simulink library "HEMERO"  (Simulink 3.00)
values from neighbouring files (symbols this model uses):
  K1 = 0.5    [ejh64.m]    (also in ejh65.m)
  K2 = 0.8    [ejh64.m]    (also in ejh65.m)
  x_camino = 0:0.01:10    [ejh64.m]    (also in ejh65.m)
  y_camino = x_camino.^2    [ejh64.m]    (also in ejh65.m)
undefined symbols (not defined in the file or in its folder): magnitude, nonlinear
libraries: simulink_extras x12, HEMERO x9, simulink3 x6, dspstat x4
(part 5 of 9)

== system HEMERO/Robots móviles/Control de robots móviles/Métodos basados en Teoría de Control/Seguimiento de caminos/Seguimiento de caminos (control lineal)/Convertidor ==
  R_c : Inport  Port=1  PortWidth=-1  SampleTime=-1  DataType=auto
      settings: SignalType=auto
  fi_gorro : Inport  Port=2  PortWidth=-1  SampleTime=-1  DataType=auto
      settings: SignalType=auto
  v : Inport  Port=3  PortWidth=-1  SampleTime=-1  DataType=auto
      settings: SignalType=auto
  u_cont : Inport  Port=4  PortWidth=-1  SampleTime=-1  DataType=auto
      settings: SignalType=auto
  Constant : Constant  Value=1
  Gain : Gain  Gain=-1  SaturateOnIntegerOverflow=on
  Math Function : Math  Operator=reciprocal  OutputSignalType=auto
  Math Function1 : Math  Operator=reciprocal  OutputSignalType=auto
  Product : Product  Inputs=3  SaturateOnIntegerOverflow=on
  Product1 : Product  Inputs=3  SaturateOnIntegerOverflow=on
  Product2 : Product  Inputs=2  SaturateOnIntegerOverflow=on
  Sum : Sum  Inputs=++  SaturateOnIntegerOverflow=on
  Sum1 : Sum  Inputs=++  SaturateOnIntegerOverflow=on
  Trigonometric Function : Trigonometry  Operator=cos  OutputSignalType=auto
  Trigonometric Function1 : Trigonometry  Operator=sin  OutputSignalType=auto
  w : Outport  Port=1  InitialOutput=0
  wires:
  Product2/1 -> Product/3
  Sum/1 -> w/1
  u_cont/1 -> Sum/1
  Product/1 -> Sum/2
  Math Function/1 -> Product2/1
  v/1 -> Product/2, Product1/2
  Trigonometric Function/1 -> Product/1
  Sum1/1 -> Math Function/1
  Constant/1 -> Sum1/2
  Product1/1 -> Sum1/1
  Gain/1 -> Product1/3
  Trigonometric Function1/1 -> Product1/1
  fi_gorro/1 -> Trigonometric Function1/1, Trigonometric Function/1
  R_c/1 -> Math Function1/1
  Math Function1/1 -> Product2/2, Gain/1

== system HEMERO/Robots móviles/Control de robots móviles/Métodos basados en Teoría de Control/Seguimiento de caminos/Seguimiento de caminos (control lineal)/Cálculo de parámetros ==
  x_camino : Inport  Port=1  PortWidth=-1  SampleTime=-1  DataType=auto
      settings: SignalType=auto
  y_camino : Inport  Port=2  PortWidth=-1  SampleTime=-1  DataType=auto
      settings: SignalType=auto
  x_vehiculo : Inport  Port=3  PortWidth=-1  SampleTime=-1  DataType=auto
      settings: SignalType=auto
  y_vehiculo : Inport  Port=4  PortWidth=-1  SampleTime=-1  DataType=auto
      settings: SignalType=auto
  phi_vehiculo : Inport  Port=5  PortWidth=-1  SampleTime=-1  DataType=auto
      settings: SignalType=auto
  Cálculo de phi gorro : Subsystem
  Degrees to Radians : simulink_extras/Transformations/Degrees to Radians
  Subsystem : Subsystem
  epsilon : Outport  Port=1
  fi_gorro : Outport  Port=2
  R_c : Outport  Port=3
  wires:
  Subsystem/2(indice) -> Cálculo de phi gorro/2(indice)
  Subsystem/1(distancia) -> epsilon/1
  Cálculo de phi gorro/1(fi_go_mo) -> Degrees to Radians/1
  Degrees to Radians/1 -> fi_gorro/1
  phi_vehiculo/1 -> Cálculo de phi gorro/1(fi_vehiculo)
  Subsystem/3(R_c) -> R_c/1
  x_vehiculo/1 -> Subsystem/3(x_vehiculo)
  y_vehiculo/1 -> Subsystem/4(y_vehiculo)
  y_camino/1 -> Subsystem/2(y_camino)
  x_camino/1 -> Subsystem/1(x_camino)

== system HEMERO/Robots móviles/Control de robots móviles/Métodos basados en Teoría de Control/Seguimiento de caminos/Seguimiento de caminos (control no lineal)/  ==
  v : Inport  Port=1  PortWidth=-1  SampleTime=-1  DataType=auto
      settings: SignalType=auto
  Abs : Abs
  Gain : Gain  Gain=K2  SaturateOnIntegerOverflow=on
  k (v) : Outport  Port=1
  wires:
  Gain/1 -> k (v)/1
  Abs/1 -> Gain/1
  v/1 -> Abs/1

== system HEMERO/Robots móviles/Control de robots móviles/Métodos basados en Teoría de Control/Seguimiento de caminos/Seguimiento de caminos (control no lineal)/Configuracion síncrona ==
  v : Inport  Port=1  PortWidth=-1  SampleTime=-1  DataType=auto
      settings: SignalType=auto
  w : Inport  Port=2  PortWidth=-1  SampleTime=-1  DataType=auto
      settings: SignalType=auto
  Fcn : Fcn  Expr=-sin(u)
  Fcn1 : Fcn  Expr=cos(u)
  Integrator : Integrator  ExternalReset=none  InitialConditionSource=internal  InitialCondition=phi_inicial  LimitOutput=off  UpperSaturationLimit=inf  LowerSaturationLimit=-inf  ShowSaturationPort=off  ShowStatePort=off  AbsoluteTolerance=auto
  Integrator1 : Integrator  ExternalReset=none  InitialConditionSource=internal  InitialCondition=x_inicial  LimitOutput=off  UpperSaturationLimit=inf  LowerSaturationLimit=-inf  ShowSaturationPort=off  ShowStatePort=off  AbsoluteTolerance=auto
  Integrator2 : Integrator  ExternalReset=none  InitialConditionSource=internal  InitialCondition=y_inicial  LimitOutput=off  UpperSaturationLimit=inf  LowerSaturationLimit=-inf  ShowSaturationPort=off  ShowStatePort=off  AbsoluteTolerance=auto
  Product : Product  Inputs=2  SaturateOnIntegerOverflow=on
  Product1 : Product  Inputs=2  SaturateOnIntegerOverflow=on
  x_vehículo : Outport  Port=1
  y_vehículo : Outport  Port=2
  phi_vehículo : Outport  Port=3
  wires:
  Fcn1/1 -> Product1/2
  w/1 -> Integrator/1
  v/1 -> Product1/1, Product/1
  Integrator2/1 -> y_vehículo/1
  Integrator1/1 -> x_vehículo/1
  Integrator/1 -> phi_vehículo/1, Fcn1/1, Fcn/1
  Fcn/1 -> Product/2
  Product/1 -> Integrator1/1
  Product1/1 -> Integrator2/1

== system HEMERO/Robots móviles/Control de robots móviles/Métodos basados en Teoría de Control/Seguimiento de caminos/Seguimiento de caminos (control no lineal)/Controlador no lineal ==
  phi_gorro : Inport  Port=1  PortWidth=-1  SampleTime=-1  DataType=auto
      settings: SignalType=auto
  v : Inport  Port=2  PortWidth=-1  SampleTime=-1  DataType=auto
      settings: SignalType=auto
  epsilon : Inport  Port=3  PortWidth=-1  SampleTime=-1  DataType=auto
      settings: SignalType=auto
  k (v) : Inport  Port=4  PortWidth=-1  SampleTime=-1  DataType=auto
      settings: SignalType=auto
  Gain : Gain  Gain=K1  SaturateOnIntegerOverflow=on
  MATLAB Fcn : MATLABFcn  MATLABFcn=nonlinear(u)  OutputWidth=-1  OutputSignalType=auto
  Product : Product  Inputs=3  SaturateOnIntegerOverflow=on
  Product1 : Product  Inputs=2  SaturateOnIntegerOverflow=on
  Sum : Sum  Inputs=--  SaturateOnIntegerOverflow=on
  u_cont : Outport  Port=1  InitialOutput=0
  wires:
  k (v)/1 -> Product1/2
  v/1 -> Product/2
  phi_gorro/1 -> Product1/1, MATLAB Fcn/1
  Gain/1 -> Product/1
  Product/1 -> Sum/1
  Product1/1 -> Sum/2
  epsilon/1 -> Gain/1
  Sum/1 -> u_cont/1
  MATLAB Fcn/1 -> Product/3

== system HEMERO/Robots móviles/Control de robots móviles/Métodos basados en Teoría de Control/Seguimiento de caminos/Seguimiento de caminos (control no lineal)/Convertidor ==
  R_c : Inport  Port=1  PortWidth=-1  SampleTime=-1  DataType=auto
      settings: SignalType=auto
  fi_gorro : Inport  Port=2  PortWidth=-1  SampleTime=-1  DataType=auto
      settings: SignalType=auto
  v : Inport  Port=3  PortWidth=-1  SampleTime=-1  DataType=auto
      settings: SignalType=auto
  u_cont : Inport  Port=4  PortWidth=-1  SampleTime=-1  DataType=auto
      settings: SignalType=auto
  Constant : Constant  Value=1
  Gain : Gain  Gain=-1  SaturateOnIntegerOverflow=on
  Math Function : Math  Operator=reciprocal  OutputSignalType=auto
  Math Function1 : Math  Operator=reciprocal  OutputSignalType=auto
  Product : Product  Inputs=3  SaturateOnIntegerOverflow=on
  Product1 : Product  Inputs=3  SaturateOnIntegerOverflow=on
  Product2 : Product  Inputs=2  SaturateOnIntegerOverflow=on
  Sum : Sum  Inputs=++  SaturateOnIntegerOverflow=on
  Sum1 : Sum  Inputs=++  SaturateOnIntegerOverflow=on
  Trigonometric Function : Trigonometry  Operator=cos  OutputSignalType=auto
  Trigonometric Function1 : Trigonometry  Operator=sin  OutputSignalType=auto
  w : Outport  Port=1  InitialOutput=0
  wires:
  Math Function1/1 -> Gain/1, Product2/2
  R_c/1 -> Math Function1/1
  fi_gorro/1 -> Trigonometric Function/1, Trigonometric Function1/1
  Trigonometric Function1/1 -> Product1/1
  Gain/1 -> Product1/3
  Product1/1 -> Sum1/1
  Constant/1 -> Sum1/2
  Sum1/1 -> Math Function/1
  Trigonometric Function/1 -> Product/1
  v/1 -> Product1/2, Product/2
  Math Function/1 -> Product2/1
  Product/1 -> Sum/2
  u_cont/1 -> Sum/1
  Sum/1 -> w/1
  Product2/1 -> Product/3

== system HEMERO/Robots móviles/Control de robots móviles/Métodos basados en Teoría de Control/Seguimiento de caminos/Seguimiento de caminos (control no lineal)/Cálculo de parámetros ==
  x_camino : Inport  Port=1  PortWidth=-1  SampleTime=-1  DataType=auto
      settings: SignalType=auto
  y_camino : Inport  Port=2  PortWidth=-1  SampleTime=-1  DataType=auto
      settings: SignalType=auto
  x_vehiculo : Inport  Port=3  PortWidth=-1  SampleTime=-1  DataType=auto
      settings: SignalType=auto
  y_vehiculo : Inport  Port=4  PortWidth=-1  SampleTime=-1  DataType=auto
      settings: SignalType=auto
  phi_vehiculo : Inport  Port=5  PortWidth=-1  SampleTime=-1  DataType=auto
      settings: SignalType=auto
  Cálculo de phi gorro : Subsystem
  Degrees to Radians : simulink_extras/Transformations/Degrees to Radians
  Subsystem : Subsystem
  epsilon : Outport  Port=1
  fi_gorro : Outport  Port=2
  R_c : Outport  Port=3
  wires:
  x_camino/1 -> Subsystem/1(x_camino)
  y_camino/1 -> Subsystem/2(y_camino)
  y_vehiculo/1 -> Subsystem/4(y_vehiculo)
  x_vehiculo/1 -> Subsystem/3(x_vehiculo)
  Subsystem/3(R_c) -> R_c/1
  phi_vehiculo/1 -> Cálculo de phi gorro/1(fi_vehiculo)
  Degrees to Radians/1 -> fi_gorro/1
  Cálculo de phi gorro/1(fi_go_mo) -> Degrees to Radians/1
  Subsystem/1(distancia) -> epsilon/1
  Subsystem/2(indice) -> Cálculo de phi gorro/2(indice)

== system HEMERO/Robots móviles/Control de robots móviles/Métodos basados en Teoría de Control/Seguimiento de trayectorias/Ejemplos/Ejemplo H.6.6 ==
  Seguimiento de trayectorias (Control lineal) : Subsystem  mask(Seguimiento de trayectorias empleando una ley de control lineal){K1=1, K2=2, K3=4, x_inicial=1, y_inicial=0.5, phi_inicial=pi/6, x_r_inicial=0, y_r_inicial=0, phi_r_inicial=0}
      mask prompts: K1 "Parámetro K1:"; K2 "Parámetro K2:"; K3 "Parámetro K3:"; x_inicial "Coordenada x inicial del robot:"; y_inicial "Coordenada y inicial del robot:"; phi_inicial "Valor inicial de la orientación del robot (rad):"; x_r_inicial "Coordenada x inicial de la referencia:"; y_r_inicial "Coordenada y inicial de la referencia:"; phi_r_inicial "Orientación inicial de la referencia (rad):"
      mask help:
      | Este bloque permite simular una estrategia de control lineal para el seguimiento de trayectorias. A la entrada se dispone de las velocidades lineal y angular de referencia. Se supone un cierto modelo para el vehículo.
      | El usuario puede modificar fácilmente este bloque para introducir como referencia las coordenadas (x,y) y la orientación deseadas.
  Step : Step  Time=0  Before=0  After=0.2  SampleTime=0
  Step1 : Step  Time=0  Before=0  After=0.3  SampleTime=0
  Step2 : Step  Time=20  Before=0  After=-0.1  SampleTime=0
  Step3 : Step  Time=10  Before=0  After=-0.1  SampleTime=0
  Sum : Sum  Inputs=++  SaturateOnIntegerOverflow=on
  Sum1 : Sum  Inputs=++  SaturateOnIntegerOverflow=on
  To Workspace : ToWorkspace  VariableName=v  SampleTime=-1  SaveFormat=Matrix
  To Workspace1 : ToWorkspace  VariableName=w  SampleTime=-1  SaveFormat=Matrix
  To Workspace2 : ToWorkspace  VariableName=v_r  SampleTime=-1  SaveFormat=Matrix
  To Workspace3 : ToWorkspace  VariableName=w_r  SampleTime=-1  SaveFormat=Matrix
  To Workspace4 : ToWorkspace  VariableName=x_r  SampleTime=-1  SaveFormat=Matrix
  To Workspace5 : ToWorkspace  VariableName=x  SampleTime=-1  SaveFormat=Matrix
  To Workspace6 : ToWorkspace  VariableName=y_r  SampleTime=-1  SaveFormat=Matrix
  To Workspace7 : ToWorkspace  VariableName=y  SampleTime=-1  SaveFormat=Matrix
  To Workspace8 : ToWorkspace  VariableName=phi_r  SampleTime=-1  SaveFormat=Matrix
  To Workspace9 : ToWorkspace  VariableName=phi  SampleTime=-1  SaveFormat=Matrix
  wires:
  Step2/1 -> Sum/1
  Step/1 -> Sum/2
  Step1/1 -> Sum1/1
  Step3/1 -> Sum1/2
  Sum1/1 -> To Workspace3/1, Seguimiento de trayectorias (Control lineal)/2(w_r)
  Sum/1 -> To Workspace2/1, Seguimiento de trayectorias (Control lineal)/1(v_r)
  Seguimiento de trayectorias (Control lineal)/1(v) -> To Workspace/1
  Seguimiento de trayectorias (Control lineal)/2(w) -> To Workspace1/1
  Seguimiento de trayectorias (Control lineal)/3(x_ref) -> To Workspace4/1
  Seguimiento de trayectorias (Control lineal)/5(y_ref) -> To Workspace6/1
  Seguimiento de trayectorias (Control lineal)/6(y) -> To Workspace7/1
  Seguimiento de trayectorias (Control lineal)/7(phi_ref) -> To Workspace8/1
  Seguimiento de trayectorias (Control lineal)/4(x) -> To Workspace5/1
  Seguimiento de trayectorias (Control lineal)/8(phi) -> To Workspace9/1

== system HEMERO/Robots móviles/Control de robots móviles/Métodos basados en Teoría de Control/Seguimiento de trayectorias/Ejemplos/Ejemplo H.6.7 ==
  Seguimiento de trayectorias (Control lineal con escalado de velocidad) : Subsystem  mask(Seguimiento de trayectorias (control lineal y escalado en velocidad)){b=13.75, d=0.9, x_inicial=1, y_inicial=0.5, phi_inicial=pi/6, x_r_inicial=0, y_r_inicial=0, phi_r_inicial=0}
      mask prompts: b "Parámetro beta:"; d "Parámetro delta:"; x_inicial "Coordenada x inicial del robot:"; y_inicial "Coordenada y inicial del robot:"; phi_inicial "Valor inicial de la orientación del robot (rad):"; x_r_inicial "Coordenada x inicial de la referencia:"; y_r_inicial "Coordenada y inicial de la referencia:"; phi_r_inicial "Orientación inicial de la referencia (rad):"
      mask help:
      | Este bloque permite simular una estrategia de control lineal con "escalado en velocidad" para el seguimiento de trayectorias. A la entrada se dispone de las velocidades lineal y angular de referencia. Se supone un cierto modelo para el vehículo.
      | El usuario puede modificar fácilmente este bloque para introducir como referencia las coordenadas (x,y) y la orientación deseadas.
  Step : Step  Time=0  Before=0  After=0.2  SampleTime=0
  Step1 : Step  Time=0  Before=0  After=0.3  SampleTime=0
  Step2 : Step  Time=20  Before=0  After=-0.1  SampleTime=0
  Step3 : Step  Time=10  Before=0  After=-0.1  SampleTime=0
  Sum : Sum  Inputs=++  SaturateOnIntegerOverflow=on
  Sum1 : Sum  Inputs=++  SaturateOnIntegerOverflow=on
  To Workspace : ToWorkspace  VariableName=v  SampleTime=-1  SaveFormat=Matrix
  To Workspace1 : ToWorkspace  VariableName=w  SampleTime=-1  SaveFormat=Matrix
  To Workspace2 : ToWorkspace  VariableName=v_r  SampleTime=-1  SaveFormat=Matrix
  To Workspace3 : ToWorkspace  VariableName=w_r  SampleTime=-1  SaveFormat=Matrix
  To Workspace4 : ToWorkspace  VariableName=x_r  SampleTime=-1  SaveFormat=Matrix
  To Workspace5 : ToWorkspace  VariableName=x  SampleTime=-1  SaveFormat=Matrix
  To Workspace6 : ToWorkspace  VariableName=y_r  SampleTime=-1  SaveFormat=Matrix
  To Workspace7 : ToWorkspace  VariableName=y  SampleTime=-1  SaveFormat=Matrix
  To Workspace8 : ToWorkspace  VariableName=phi_r  SampleTime=-1  SaveFormat=Matrix
  To Workspace9 : ToWorkspace  VariableName=phi  SampleTime=-1  SaveFormat=Matrix
  wires:
  Step2/1 -> Sum/1
  Step/1 -> Sum/2
  Step1/1 -> Sum1/1
  Step3/1 -> Sum1/2
  Sum1/1 -> To Workspace3/1, Seguimiento de trayectorias (Control lineal con escalado de velocidad)/2(w_r)
  Sum/1 -> To Workspace2/1, Seguimiento de trayectorias (Control lineal con escalado de velocidad)/1(v_r)
  Seguimiento de trayectorias (Control lineal con escalado de velocidad)/1(v) -> To Workspace/1
  Seguimiento de trayectorias (Control lineal con escalado de velocidad)/2(w) -> To Workspace1/1
  Seguimiento de trayectorias (Control lineal con escalado de velocidad)/3(x_ref) -> To Workspace4/1
  Seguimiento de trayectorias (Control lineal con escalado de velocidad)/5(y_ref) -> To Workspace6/1
  Seguimiento de trayectorias (Control lineal con escalado de velocidad)/6(y) -> To Workspace7/1
  Seguimiento de trayectorias (Control lineal con escalado de velocidad)/7(phi_ref) -> To Workspace8/1
  Seguimiento de trayectorias (Control lineal con escalado de velocidad)/4(x) -> To Workspace5/1
  Seguimiento de trayectorias (Control lineal con escalado de velocidad)/8(phi) -> To Workspace9/1

== system HEMERO/Robots móviles/Control de robots móviles/Métodos basados en Teoría de Control/Seguimiento de trayectorias/Ejemplos/Ejemplo H.6.8 ==
  Seguimiento de trayectorias (Control no lineal) : Subsystem  mask(Seguimiento de trayectorias empleando una ley de control no lineal){b=13.75, d=0.9, K2=19, x_inicial=1, y_inicial=0.5, phi_inicial=pi/6, x_r_inicial=0, y_r_inicial=0, phi_r_inicial=0}
      mask prompts: b "Parámetro beta:"; d "Parámetro delta:"; K2 "Parámetro K2:"; x_inicial "Coordenada x inicial del robot:"; y_inicial "Coordenada y inicial del robot:"; phi_inicial "Valor inicial de la orientación del robot (rad):"; x_r_inicial "Coordenada x inicial de la referencia:"; y_r_inicial "Coordenada y inicial de la referencia:"; phi_r_inicial "Orientación inicial de la referencia (rad):"
      mask help:
      | Este bloque permite simular una estrategia de control no lineal para el seguimiento de trayectorias. A la entrada se dispone de las velocidades lineal y angular de referencia. Se supone un cierto modelo para el vehículo.
      | El usuario puede modificar este bloque para introducir como referencia las coordenadas (x,y) y la orientación deseadas.
  Step : Step  Time=0  Before=0  After=0.2  SampleTime=0
  Step1 : Step  Time=0  Before=0  After=0.3  SampleTime=0
  Step2 : Step  Time=20  Before=0  After=-0.1  SampleTime=0
  Step3 : Step  Time=10  Before=0  After=-0.1  SampleTime=0
  Sum : Sum  Inputs=++  SaturateOnIntegerOverflow=on
  Sum1 : Sum  Inputs=++  SaturateOnIntegerOverflow=on
  To Workspace : ToWorkspace  VariableName=v  SampleTime=-1  SaveFormat=Matrix
  To Workspace1 : ToWorkspace  VariableName=w  SampleTime=-1  SaveFormat=Matrix
  To Workspace2 : ToWorkspace  VariableName=v_r  SampleTime=-1  SaveFormat=Matrix
  To Workspace3 : ToWorkspace  VariableName=w_r  SampleTime=-1  SaveFormat=Matrix
  To Workspace4 : ToWorkspace  VariableName=x_r  SampleTime=-1  SaveFormat=Matrix
  To Workspace5 : ToWorkspace  VariableName=x  SampleTime=-1  SaveFormat=Matrix
  To Workspace6 : ToWorkspace  VariableName=y_r  SampleTime=-1  SaveFormat=Matrix
  To Workspace7 : ToWorkspace  VariableName=y  SampleTime=-1  SaveFormat=Matrix
  To Workspace8 : ToWorkspace  VariableName=phi_r  SampleTime=-1  SaveFormat=Matrix
  To Workspace9 : ToWorkspace  VariableName=phi  SampleTime=-1  SaveFormat=Matrix
  wires:
  Step2/1 -> Sum/1
  Step/1 -> Sum/2
  Step1/1 -> Sum1/1
  Step3/1 -> Sum1/2
  Sum1/1 -> To Workspace3/1, Seguimiento de trayectorias (Control no lineal)/2(w_r)
  Sum/1 -> To Workspace2/1, Seguimiento de trayectorias (Control no lineal)/1(v_r)
  Seguimiento de trayectorias (Control no lineal)/1(v) -> To Workspace/1
  Seguimiento de trayectorias (Control no lineal)/2(w) -> To Workspace1/1
  Seguimiento de trayectorias (Control no lineal)/3(x_ref) -> To Workspace4/1
  Seguimiento de trayectorias (Control no lineal)/5(y_ref) -> To Workspace6/1
  Seguimiento de trayectorias (Control no lineal)/6(y) -> To Workspace7/1
  Seguimiento de trayectorias (Control no lineal)/7(phi_ref) -> To Workspace8/1
  Seguimiento de trayectorias (Control no lineal)/4(x) -> To Workspace5/1
  Seguimiento de trayectorias (Control no lineal)/8(phi) -> To Workspace9/1

== system HEMERO/Robots móviles/Control de robots móviles/Métodos basados en Teoría de Control/Seguimiento de trayectorias/Seguimiento de trayectorias (Control lineal con escalado de velocidad)/Cambio de variable ==
  x_r : Inport  Port=1  PortWidth=-1  SampleTime=-1  DataType=auto
      settings: SignalType=auto
  x : Inport  Port=2  PortWidth=-1  SampleTime=-1  DataType=auto
      settings: SignalType=auto
  y_r : Inport  Port=3  PortWidth=-1  SampleTime=-1  DataType=auto
      settings: SignalType=auto
  y : Inport  Port=4  PortWidth=-1  SampleTime=-1  DataType=auto
      settings: SignalType=auto
  phi_r : Inport  Port=5  PortWidth=-1  SampleTime=-1  DataType=auto
      settings: SignalType=auto
  phi : Inport  Port=6  PortWidth=-1  SampleTime=-1  DataType=auto
      settings: SignalType=auto
  Cálculo de e1 : Subsystem
  Cálculo de e2 : Subsystem
  Cálculo de e3 : Subsystem
  e1 : Outport  Port=1
  e2 : Outport  Port=2
  e3 : Outport  Port=3
  wires:
  Cálculo de e3/1(e3) -> e3/1
  Cálculo de e2/1(e2) -> e2/1
  Cálculo de e1/1(e1) -> e1/1
  phi/1 -> Cálculo de e1/5(phi), Cálculo de e3/2(phi), Cálculo de e2/5(phi)
  phi_r/1 -> Cálculo de e3/1(phi_r)
  y/1 -> Cálculo de e2/4(y), Cálculo de e1/4(y)
  y_r/1 -> Cálculo de e2/3(y_r), Cálculo de e1/3(y_r)
  x/1 -> Cálculo de e2/2(x), Cálculo de e1/2(x)
  x_r/1 -> Cálculo de e2/1(x_r), Cálculo de e1/1(x_r)

== system HEMERO/Robots móviles/Control de robots móviles/Métodos basados en Teoría de Control/Seguimiento de trayectorias/Seguimiento de trayectorias (Control lineal con escalado de velocidad)/Configuración síncrona referencia ==
  v_r : Inport  Port=1  PortWidth=-1  SampleTime=-1  DataType=auto
      settings: SignalType=auto
  w_r : Inport  Port=2  PortWidth=-1  SampleTime=-1  DataType=auto
      settings: SignalType=auto
  Gain : Gain  Gain=-1  SaturateOnIntegerOverflow=on
  Integrator : Integrator  ExternalReset=none  InitialConditionSource=internal  InitialCondition=phi_r_inicial  LimitOutput=off  UpperSaturationLimit=inf  LowerSaturationLimit=-inf  ShowSaturationPort=off  ShowStatePort=off  AbsoluteTolerance=auto
  Integrator1 : Integrator  ExternalReset=none  InitialConditionSource=internal  InitialCondition=x_r_inicial  LimitOutput=off  UpperSaturationLimit=inf  LowerSaturationLimit=-inf  ShowSaturationPort=off  ShowStatePort=off  AbsoluteTolerance=auto
  Integrator2 : Integrator  ExternalReset=none  InitialConditionSource=internal  InitialCondition=y_r_inicial  LimitOutput=off  UpperSaturationLimit=inf  LowerSaturationLimit=-inf  ShowSaturationPort=off  ShowStatePort=off  AbsoluteTolerance=auto
  Product : Product  Inputs=2  SaturateOnIntegerOverflow=on
  Product1 : Product  Inputs=2  SaturateOnIntegerOverflow=on
  Trigonometric Function : Trigonometry  Operator=sin  OutputSignalType=auto
  Trigonometric Function1 : Trigonometry  Operator=cos  OutputSignalType=auto
  x_r : Outport  Port=1
  y_r : Outport  Port=2
  phi_r : Outport  Port=3
  wires:
  Trigonometric Function1/1 -> Product1/2
  Trigonometric Function/1 -> Gain/1
  w_r/1 -> Integrator/1
  v_r/1 -> Product1/1, Product/1
  Integrator2/1 -> y_r/1
  Integrator1/1 -> x_r/1
  Integrator/1 -> phi_r/1, Trigonometric Function1/1, Trigonometric Function/1
  Gain/1 -> Product/2
  Product/1 -> Integrator1/1
  Product1/1 -> Integrator2/1

== system HEMERO/Robots móviles/Control de robots móviles/Métodos basados en Teoría de Control/Seguimiento de trayectorias/Seguimiento de trayectorias (Control lineal con escalado de velocidad)/Configuración síncrona robot real ==
  v : Inport  Port=1  PortWidth=-1  SampleTime=-1  DataType=auto
      settings: SignalType=auto
  w : Inport  Port=2  PortWidth=-1  SampleTime=-1  DataType=auto
      settings: SignalType=auto
  Gain : Gain  Gain=-1  SaturateOnIntegerOverflow=on
  Integrator : Integrator  ExternalReset=none  InitialConditionSource=internal  InitialCondition=phi_inicial  LimitOutput=off  UpperSaturationLimit=inf  LowerSaturationLimit=-inf  ShowSaturationPort=off  ShowStatePort=off  AbsoluteTolerance=auto
  Integrator1 : Integrator  ExternalReset=none  InitialConditionSource=internal  InitialCondition=x_inicial  LimitOutput=off  UpperSaturationLimit=inf  LowerSaturationLimit=-inf  ShowSaturationPort=off  ShowStatePort=off  AbsoluteTolerance=auto
  Integrator2 : Integrator  ExternalReset=none  InitialConditionSource=internal  InitialCondition=y_inicial  LimitOutput=off  UpperSaturationLimit=inf  LowerSaturationLimit=-inf  ShowSaturationPort=off  ShowStatePort=off  AbsoluteTolerance=auto
  Product : Product  Inputs=2  SaturateOnIntegerOverflow=on
  Product1 : Product  Inputs=2  SaturateOnIntegerOverflow=on
  Trigonometric Function : Trigonometry  Operator=sin  OutputSignalType=auto
  Trigonometric Function1 : Trigonometry  Operator=cos  OutputSignalType=auto
  x : Outport  Port=1
  y : Outport  Port=2
  phi : Outport  Port=3
  wires:
  Trigonometric Function1/1 -> Product1/2
  Trigonometric Function/1 -> Gain/1
  w/1 -> Integrator/1
  v/1 -> Product1/1, Product/1
  Integrator2/1 -> y/1
  Integrator1/1 -> x/1
  Integrator/1 -> phi/1, Trigonometric Function1/1, Trigonometric Function/1
  Gain/1 -> Product/2
  Product/1 -> Integrator1/1
  Product1/1 -> Integrator2/1

== system HEMERO/Robots móviles/Control de robots móviles/Métodos basados en Teoría de Control/Seguimiento de trayectorias/Seguimiento de trayectorias (Control lineal con escalado de velocidad)/Control lineal con escalado de velocidad ==
  e1 : Inport  Port=1  PortWidth=-1  SampleTime=-1  DataType=auto
      settings: SignalType=auto
  e2 : Inport  Port=2  PortWidth=-1  SampleTime=-1  DataType=auto
      settings: SignalType=auto
  e3 : Inport  Port=3  PortWidth=-1  SampleTime=-1  DataType=auto
      settings: SignalType=auto
  v_r : Inport  Port=4  PortWidth=-1  SampleTime=-1  DataType=auto
      settings: SignalType=auto
  w_r : Inport  Port=5  PortWidth=-1  SampleTime=-1  DataType=auto
      settings: SignalType=auto
  Cálculo de u1 : Subsystem
  "Cálculo de u2 " : Subsystem
  u1 : Outport  Port=1
  u2 : Outport  Port=2
  wires:
  Cálculo de u1/2(K1) -> "Cálculo de u2 "/4(K3)
  w_r/1 -> Cálculo de u1/3(w_r)
  "Cálculo de u2 "/1(u2) -> u2/1
  Cálculo de u1/1(u1) -> u1/1
  e3/1 -> "Cálculo de u2 "/2(e3)
  e2/1 -> "Cálculo de u2 "/1(e2)
  v_r/1 -> "Cálculo de u2 "/3(v_r), Cálculo de u1/2(v_r)
  e1/1 -> Cálculo de u1/1(e1)

== system HEMERO/Robots móviles/Control de robots móviles/Métodos basados en Teoría de Control/Seguimiento de trayectorias/Seguimiento de trayectorias (Control lineal)/Cambio de variable ==
  x_r : Inport  Port=1  PortWidth=-1  SampleTime=-1  DataType=auto
      settings: SignalType=auto
  x : Inport  Port=2  PortWidth=-1  SampleTime=-1  DataType=auto
      settings: SignalType=auto
  y_r : Inport  Port=3  PortWidth=-1  SampleTime=-1  DataType=auto
      settings: SignalType=auto
  y : Inport  Port=4  PortWidth=-1  SampleTime=-1  DataType=auto
      settings: SignalType=auto
  phi_r : Inport  Port=5  PortWidth=-1  SampleTime=-1  DataType=auto
      settings: SignalType=auto
  phi : Inport  Port=6  PortWidth=-1  SampleTime=-1  DataType=auto
      settings: SignalType=auto
  Cálculo de e1 : Subsystem
  Cálculo de e2 : Subsystem
  Cálculo de e3 : Subsystem
  e1 : Outport  Port=1
  e2 : Outport  Port=2
  e3 : Outport  Port=3
  wires:
  Cálculo de e3/1(e3) -> e3/1
  Cálculo de e2/1(e2) -> e2/1
  Cálculo de e1/1(e1) -> e1/1
  phi/1 -> Cálculo de e1/5(phi), Cálculo de e3/2(phi), Cálculo de e2/5(phi)
  phi_r/1 -> Cálculo de e3/1(phi_r)
  y/1 -> Cálculo de e2/4(y), Cálculo de e1/4(y)
  y_r/1 -> Cálculo de e2/3(y_r), Cálculo de e1/3(y_r)
  x/1 -> Cálculo de e2/2(x), Cálculo de e1/2(x)
  x_r/1 -> Cálculo de e2/1(x_r), Cálculo de e1/1(x_r)

== system HEMERO/Robots móviles/Control de robots móviles/Métodos basados en Teoría de Control/Seguimiento de trayectorias/Seguimiento de trayectorias (Control lineal)/Configuración síncrona referencia ==
  v_r : Inport  Port=1  PortWidth=-1  SampleTime=-1  DataType=auto
      settings: SignalType=auto
  w_r : Inport  Port=2  PortWidth=-1  SampleTime=-1  DataType=auto
      settings: SignalType=auto
  Gain : Gain  Gain=-1  SaturateOnIntegerOverflow=on
  Integrator : Integrator  ExternalReset=none  InitialConditionSource=internal  InitialCondition=phi_r_inicial  LimitOutput=off  UpperSaturationLimit=inf  LowerSaturationLimit=-inf  ShowSaturationPort=off  ShowStatePort=off  AbsoluteTolerance=auto
  Integrator1 : Integrator  ExternalReset=none  InitialConditionSource=internal  InitialCondition=x_r_inicial  LimitOutput=off  UpperSaturationLimit=inf  LowerSaturationLimit=-inf  ShowSaturationPort=off  ShowStatePort=off  AbsoluteTolerance=auto
  Integrator2 : Integrator  ExternalReset=none  InitialConditionSource=internal  InitialCondition=y_r_inicial  LimitOutput=off  UpperSaturationLimit=inf  LowerSaturationLimit=-inf  ShowSaturationPort=off  ShowStatePort=off  AbsoluteTolerance=auto
  Product : Product  Inputs=2  SaturateOnIntegerOverflow=on
  Product1 : Product  Inputs=2  SaturateOnIntegerOverflow=on
  Trigonometric Function : Trigonometry  Operator=sin  OutputSignalType=auto
  Trigonometric Function1 : Trigonometry  Operator=cos  OutputSignalType=auto
  x_r : Outport  Port=1
  y_r : Outport  Port=2
  phi_r : Outport  Port=3
  wires:
  Gain/1 -> Product/2
  Trigonometric Function/1 -> Gain/1
  w_r/1 -> Integrator/1
  v_r/1 -> Product1/1, Product/1
  Integrator2/1 -> y_r/1
  Integrator1/1 -> x_r/1
  Integrator/1 -> phi_r/1, Trigonometric Function/1, Trigonometric Function1/1
  Trigonometric Function1/1 -> Product1/2
  Product/1 -> Integrator1/1
  Product1/1 -> Integrator2/1

== system HEMERO/Robots móviles/Control de robots móviles/Métodos basados en Teoría de Control/Seguimiento de trayectorias/Seguimiento de trayectorias (Control lineal)/Configuración síncrona robot real ==
  v : Inport  Port=1  PortWidth=-1  SampleTime=-1  DataType=auto
      settings: SignalType=auto
  w : Inport  Port=2  PortWidth=-1  SampleTime=-1  DataType=auto
      settings: SignalType=auto
  Gain : Gain  Gain=-1  SaturateOnIntegerOverflow=on
  Integrator : Integrator  ExternalReset=none  InitialConditionSource=internal  InitialCondition=phi_inicial  LimitOutput=off  UpperSaturationLimit=inf  LowerSaturationLimit=-inf  ShowSaturationPort=off  ShowStatePort=off  AbsoluteTolerance=auto
  Integrator1 : Integrator  ExternalReset=none  InitialConditionSource=internal  InitialCondition=x_inicial  LimitOutput=off  UpperSaturationLimit=inf  LowerSaturationLimit=-inf  ShowSaturationPort=off  ShowStatePort=off  AbsoluteTolerance=auto
  Integrator2 : Integrator  ExternalReset=none  InitialConditionSource=internal  InitialCondition=y_inicial  LimitOutput=off  UpperSaturationLimit=inf  LowerSaturationLimit=-inf  ShowSaturationPort=off  ShowStatePort=off  AbsoluteTolerance=auto
  Product : Product  Inputs=2  SaturateOnIntegerOverflow=on
  Product1 : Product  Inputs=2  SaturateOnIntegerOverflow=on
  Trigonometric Function : Trigonometry  Operator=sin  OutputSignalType=auto
  Trigonometric Function1 : Trigonometry  Operator=cos  OutputSignalType=auto
  x : Outport  Port=1
  y : Outport  Port=2
  phi : Outport  Port=3
  wires:
  Trigonometric Function1/1 -> Product1/2
  Trigonometric Function/1 -> Gain/1
  w/1 -> Integrator/1
  v/1 -> Product1/1, Product/1
  Integrator2/1 -> y/1
  Integrator1/1 -> x/1
  Integrator/1 -> phi/1, Trigonometric Function1/1, Trigonometric Function/1
  Gain/1 -> Product/2
  Product/1 -> Integrator1/1
  Product1/1 -> Integrator2/1

== system HEMERO/Robots móviles/Control de robots móviles/Métodos basados en Teoría de Control/Seguimiento de trayectorias/Seguimiento de trayectorias (Control lineal)/Control lineal ==
  e1 : Inport  Port=1  PortWidth=-1  SampleTime=-1  DataType=auto
      settings: SignalType=auto
  e2 : Inport  Port=2  PortWidth=-1  SampleTime=-1  DataType=auto
      settings: SignalType=auto
  e3 : Inport  Port=3  PortWidth=-1  SampleTime=-1  DataType=auto
      settings: SignalType=auto
  v_r : Inport  Port=4  PortWidth=-1  SampleTime=-1  DataType=auto
      settings: SignalType=auto
  Cálculo de u1 : Subsystem
  "Cálculo de u2 " : Subsystem
  u1 : Outport  Port=1
  u2 : Outport  Port=2
  wires:
  v_r/1 -> "Cálculo de u2 "/3(v_r)
  "Cálculo de u2 "/1(u2) -> u2/1
  Cálculo de u1/1(u1) -> u1/1
  e3/1 -> "Cálculo de u2 "/2(e3)
  e2/1 -> "Cálculo de u2 "/1(e2)
  e1/1 -> Cálculo de u1/1(e1)

== system HEMERO/Robots móviles/Control de robots móviles/Métodos basados en Teoría de Control/Seguimiento de trayectorias/Seguimiento de trayectorias (Control no lineal)/Cambio de variable ==
  x_r : Inport  Port=1  PortWidth=-1  SampleTime=-1  DataType=auto
      settings: SignalType=auto
  x : Inport  Port=2  PortWidth=-1  SampleTime=-1  DataType=auto
      settings: SignalType=auto
  y_r : Inport  Port=3  PortWidth=-1  SampleTime=-1  DataType=auto
      settings: SignalType=auto
  y : Inport  Port=4  PortWidth=-1  SampleTime=-1  DataType=auto
      settings: SignalType=auto
  phi_r : Inport  Port=5  PortWidth=-1  SampleTime=-1  DataType=auto
      settings: SignalType=auto
  phi : Inport  Port=6  PortWidth=-1  SampleTime=-1  DataType=auto
      settings: SignalType=auto
  Cálculo de e1 : Subsystem
  Cálculo de e2 : Subsystem
  Cálculo de e3 : Subsystem
  e1 : Outport  Port=1
  e2 : Outport  Port=2
  e3 : Outport  Port=3
  wires:
  Cálculo de e3/1(e3) -> e3/1
  Cálculo de e2/1(e2) -> e2/1
  Cálculo de e1/1(e1) -> e1/1
  phi/1 -> Cálculo de e1/5(phi), Cálculo de e3/2(phi), Cálculo de e2/5(phi)
  phi_r/1 -> Cálculo de e3/1(phi_r)
  y/1 -> Cálculo de e2/4(y), Cálculo de e1/4(y)
  y_r/1 -> Cálculo de e2/3(y_r), Cálculo de e1/3(y_r)
  x/1 -> Cálculo de e2/2(x), Cálculo de e1/2(x)
  x_r/1 -> Cálculo de e2/1(x_r), Cálculo de e1/1(x_r)

== system HEMERO/Robots móviles/Control de robots móviles/Métodos basados en Teoría de Control/Seguimiento de trayectorias/Seguimiento de trayectorias (Control no lineal)/Configuración síncrona referencia ==
  v_r : Inport  Port=1  PortWidth=-1  SampleTime=-1  DataType=auto
      settings: SignalType=auto
  w_r : Inport  Port=2  PortWidth=-1  SampleTime=-1  DataType=auto
      settings: SignalType=auto
  Gain : Gain  Gain=-1  SaturateOnIntegerOverflow=on
  Integrator : Integrator  ExternalReset=none  InitialConditionSource=internal  InitialCondition=phi_r_inicial  LimitOutput=off  UpperSaturationLimit=inf  LowerSaturationLimit=-inf  ShowSaturationPort=off  ShowStatePort=off  AbsoluteTolerance=auto
  Integrator1 : Integrator  ExternalReset=none  InitialConditionSource=internal  InitialCondition=x_r_inicial  LimitOutput=off  UpperSaturationLimit=inf  LowerSaturationLimit=-inf  ShowSaturationPort=off  ShowStatePort=off  AbsoluteTolerance=auto
  Integrator2 : Integrator  ExternalReset=none  InitialConditionSource=internal  InitialCondition=y_r_inicial  LimitOutput=off  UpperSaturationLimit=inf  LowerSaturationLimit=-inf  ShowSaturationPort=off  ShowStatePort=off  AbsoluteTolerance=auto
  Product : Product  Inputs=2  SaturateOnIntegerOverflow=on
  Product1 : Product  Inputs=2  SaturateOnIntegerOverflow=on
  Trigonometric Function : Trigonometry  Operator=sin  OutputSignalType=auto
  Trigonometric Function1 : Trigonometry  Operator=cos  OutputSignalType=auto
  x_r : Outport  Port=1
  y_r : Outport  Port=2
  phi_r : Outport  Port=3
  wires:
  Trigonometric Function1/1 -> Product1/2
  Trigonometric Function/1 -> Gain/1
  Gain/1 -> Product/2
  w_r/1 -> Integrator/1
  v_r/1 -> Product1/1, Product/1
  Integrator2/1 -> y_r/1
  Integrator1/1 -> x_r/1
  Integrator/1 -> phi_r/1, Trigonometric Function1/1, Trigonometric Function/1
  Product/1 -> Integrator1/1
  Product1/1 -> Integrator2/1

== system HEMERO/Robots móviles/Control de robots móviles/Métodos basados en Teoría de Control/Seguimiento de trayectorias/Seguimiento de trayectorias (Control no lineal)/Configuración síncrona robot real ==
  v : Inport  Port=1  PortWidth=-1  SampleTime=-1  DataType=auto
      settings: SignalType=auto
  w : Inport  Port=2  PortWidth=-1  SampleTime=-1  DataType=auto
      settings: SignalType=auto
  Gain : Gain  Gain=-1  SaturateOnIntegerOverflow=on
  Integrator : Integrator  ExternalReset=none  InitialConditionSource=internal  InitialCondition=phi_inicial  LimitOutput=off  UpperSaturationLimit=inf  LowerSaturationLimit=-inf  ShowSaturationPort=off  ShowStatePort=off  AbsoluteTolerance=auto
  Integrator1 : Integrator  ExternalReset=none  InitialConditionSource=internal  InitialCondition=x_inicial  LimitOutput=off  UpperSaturationLimit=inf  LowerSaturationLimit=-inf  ShowSaturationPort=off  ShowStatePort=off  AbsoluteTolerance=auto
  Integrator2 : Integrator  ExternalReset=none  InitialConditionSource=internal  InitialCondition=y_inicial  LimitOutput=off  UpperSaturationLimit=inf  LowerSaturationLimit=-inf  ShowSaturationPort=off  ShowStatePort=off  AbsoluteTolerance=auto
  Product : Product  Inputs=2  SaturateOnIntegerOverflow=on
  Product1 : Product  Inputs=2  SaturateOnIntegerOverflow=on
  Trigonometric Function : Trigonometry  Operator=sin  OutputSignalType=auto
  Trigonometric Function1 : Trigonometry  Operator=cos  OutputSignalType=auto
  x : Outport  Port=1
  y : Outport  Port=2
  phi : Outport  Port=3
  wires:
  Trigonometric Function1/1 -> Product1/2
  Trigonometric Function/1 -> Gain/1
  w/1 -> Integrator/1
  v/1 -> Product1/1, Product/1
  Integrator2/1 -> y/1
  Integrator1/1 -> x/1
  Integrator/1 -> phi/1, Trigonometric Function1/1, Trigonometric Function/1
  Gain/1 -> Product/2
  Product/1 -> Integrator1/1
  Product1/1 -> Integrator2/1

== system HEMERO/Robots móviles/Control de robots móviles/Métodos basados en Teoría de Control/Seguimiento de trayectorias/Seguimiento de trayectorias (Control no lineal)/Control no lineal ==
  e1 : Inport  Port=1  PortWidth=-1  SampleTime=-1  DataType=auto
      settings: SignalType=auto
  e2 : Inport  Port=2  PortWidth=-1  SampleTime=-1  DataType=auto
      settings: SignalType=auto
  e3 : Inport  Port=3  PortWidth=-1  SampleTime=-1  DataType=auto
      settings: SignalType=auto
  v_r : Inport  Port=4  PortWidth=-1  SampleTime=-1  DataType=auto
      settings: SignalType=auto
  K1 : Inport  Port=5  PortWidth=-1  SampleTime=-1  DataType=auto
      settings: SignalType=auto
  K3 : Inport  Port=6  PortWidth=-1  SampleTime=-1  DataType=auto
      settings: SignalType=auto
  Cálculo de u1 : Subsystem
  "Cálculo de u2 " : Subsystem
  u1 : Outport  Port=1
  u2 : Outport  Port=2
  wires:
  K3/1 -> "Cálculo de u2 "/4(K3)
  K1/1 -> Cálculo de u1/2(K1)
  v_r/1 -> "Cálculo de u2 "/3(v_r)
  "Cálculo de u2 "/1(u2) -> u2/1
  Cálculo de u1/1(u1) -> u1/1
  e3/1 -> "Cálculo de u2 "/2(e3)
  e2/1 -> "Cálculo de u2 "/1(e2)
  e1/1 -> Cálculo de u1/1(e1)

== system HEMERO/Robots móviles/Control de robots móviles/Métodos basados en Teoría de Control/Seguimiento de trayectorias/Seguimiento de trayectorias (Control no lineal)/Cálculo de K1 y K3 ==
  w_r : Inport  Port=1  PortWidth=-1  SampleTime=-1  DataType=auto
      settings: SignalType=auto
  v_r : Inport  Port=2  PortWidth=-1  SampleTime=-1  DataType=auto
      settings: SignalType=auto
  Constant : Constant  Value=b
  Fcn : Fcn  Expr=u^2
  Fcn1 : Fcn  Expr=u^2
  Fcn2 : Fcn  Expr=sqrt(u)
  Gain1 : Gain  Gain=2*d  SaturateOnIntegerOverflow=on
  Product : Product  Inputs=2  SaturateOnIntegerOverflow=on
  Sum : Sum  Inputs=++  SaturateOnIntegerOverflow=on
  K1 : Outport  Port=1
  wires:
  Gain1/1 -> K1/1
  Fcn2/1 -> Gain1/1
  Sum/1 -> Fcn2/1
  Fcn/1 -> Sum/2
  Product/1 -> Sum/1
  Constant/1 -> Product/2
  Fcn1/1 -> Product/1
  v_r/1 -> Fcn1/1
  w_r/1 -> Fcn/1

== system HEMERO/Robots manipuladores base fija/Control basado en el modelo/Control con aprendizaje/Ejemplos/Ejemplo H.5.1/Par realimentado aprendido/Término de la matriz de masas estimado ==
  q : Inport  Port=1  PortWidth=-1  SampleTime=-1  DataType=auto
      settings: SignalType=auto
  In : Inport  Port=2  PortWidth=-1  SampleTime=-1  DataType=auto
      settings: SignalType=auto
  Masas : S-Function  FunctionName=sinertia  Parameters=dyn  PortCounts=[]  SFunctionModules=''
  Mux : Mux  Inputs=2
      settings: DisplayOption=none
  M (q)·In : Outport  Port=1  InitialOutput=0
  wires:
  Masas/1 -> M (q)·In/1
  In/1 -> Mux/2
  q/1 -> Mux/1
  Mux/1 -> Masas/1

== system HEMERO/Robots móviles/Control de robots móviles/Métodos basados en Teoría de Control/Seguimiento de caminos/Ejemplos/Ejemplo H.6.4/Seguimiento de caminos (control lineal) ==
  v : Inport  Port=1  PortWidth=-1  SampleTime=-1  DataType=auto
      settings: SignalType=auto
  Configuracion síncrona : Subsystem
  Constant : Constant  Value=x_camino
  Constant1 : Constant  Value=y_camino
  Controlador lineal : Subsystem  Orientation=left
  Convertidor : Subsystem  Orientation=left
      mask Description: Este bloque permite transformar la salida del controlador a una señal que será adecuada al vehículo que se desea controlar
  Cálculo de parámetros : Subsystem
  x_vehículo : Outport  Port=1
  y_vehículo : Outport  Port=2
  phi_vehículo : Outport  Port=3
  wires:
  Configuracion síncrona/3(phi_vehículo) -> phi_vehículo/1, Cálculo de parámetros/5(phi_vehiculo)
  Cálculo de parámetros/3(R_c) -> Convertidor/1(R_c)
  v/1 -> Convertidor/3(v), Controlador lineal/2(v), Configuracion síncrona/1(v)
  Configuracion síncrona/2(y_vehículo) -> y_vehículo/1, Cálculo de parámetros/4(y_vehiculo)
  Configuracion síncrona/1(x_vehículo) -> x_vehículo/1, Cálculo de parámetros/3(x_vehiculo)
  Convertidor/1(w) -> Configuracion síncrona/2(w)
  Cálculo de parámetros/1(epsilon) -> Controlador lineal/3(epsilon)
  Controlador lineal/1(u_cont) -> Convertidor/4(u_cont)
  Cálculo de parámetros/2(fi_gorro) -> Convertidor/2(fi_gorro), Controlador lineal/1(fi_gorro)
  Constant1/1 -> Cálculo de parámetros/2(y_camino)
  Constant/1 -> Cálculo de parámetros/1(x_camino)

== system HEMERO/Robots móviles/Control de robots móviles/Métodos basados en Teoría de Control/Seguimiento de caminos/Ejemplos/Ejemplo H.6.5/Seguimiento de caminos (control no lineal) ==
  v : Inport  Port=1  PortWidth=-1  SampleTime=-1  DataType=auto
      settings: SignalType=auto
  " " : Subsystem  Orientation=left  mask{K2=K2}
      mask prompts: K2 "Parámetro K2:"
  Configuracion síncrona : Subsystem
  Constant : Constant  Value=x_camino
  Constant1 : Constant  Value=y_camino
  Controlador no lineal : Subsystem  Orientation=left
  Convertidor : Subsystem  Orientation=left
      mask Description: Este bloque permite transformar la salida del controlador a una señal que será adecuada al vehículo que se desea controlar
  Cálculo de parámetros : Subsystem
  x_vehículo : Outport  Port=1
  y_vehículo : Outport  Port=2
  phi_vehículo : Outport  Port=3
  wires:
  Constant/1 -> Cálculo de parámetros/1(x_camino)
  Constant1/1 -> Cálculo de parámetros/2(y_camino)
  Cálculo de parámetros/2(fi_gorro) -> Controlador no lineal/1(phi_gorro), Convertidor/2(fi_gorro)
  Controlador no lineal/1(u_cont) -> Convertidor/4(u_cont)
  Cálculo de parámetros/1(epsilon) -> Controlador no lineal/3(epsilon)
  Configuracion síncrona/1(x_vehículo) -> Cálculo de parámetros/3(x_vehiculo), x_vehículo/1
  Configuracion síncrona/2(y_vehículo) -> Cálculo de parámetros/4(y_vehiculo), y_vehículo/1
  v/1 -> Configuracion síncrona/1(v), Convertidor/3(v), Controlador no lineal/2(v), " "/1(v)
  Cálculo de parámetros/3(R_c) -> Convertidor/1(R_c)
  " "/1(k (v)) -> Controlador no lineal/4(k (v))
  Configuracion síncrona/3(phi_vehículo) -> Cálculo de parámetros/5(phi_vehiculo), phi_vehículo/1
  Convertidor/1(w) -> Configuracion síncrona/2(w)

== system HEMERO/Robots móviles/Control de robots móviles/Métodos basados en Teoría de Control/Seguimiento de caminos/Seguimiento de caminos (control lineal)/Cálculo de parámetros/Cálculo de phi gorro ==
  fi_vehiculo : Inport  Port=1  PortWidth=-1  SampleTime=-1  DataType=auto
      settings: SignalType=auto
  indice : Inport  Port=2  PortWidth=-1  SampleTime=-1  DataType=auto
      settings: SignalType=auto
  Subsystem : Subsystem
      mask Type: Pasa phi a un ángulo entre -180 y 180
      mask Description: Pasa phi a un ángulo entre -180 y 180
      mask Help: Pasa phi a un ángulo entre -180 y 180
  Subsystem1 : Subsystem
  Subsystem2 : Subsystem
      mask Description: Pasa phi gorro al intervalo -180,180
  suma : Sum  Inputs=+-  SaturateOnIntegerOverflow=on
  fi_go_mo : Outport  Port=1
  wires:
  Subsystem1/1(fi_camino) -> suma/2
  fi_vehiculo/1 -> Subsystem/1(fi_vehiculo)
  indice/1 -> Subsystem1/1(indice)
  Subsystem/1(fi_veh_mod) -> suma/1
  suma/1 -> Subsystem2/1(fi_gorro)
  Subsystem2/1(fi_go_mo) -> fi_go_mo/1

== system HEMERO/Robots móviles/Control de robots móviles/Métodos basados en Teoría de Control/Seguimiento de caminos/Seguimiento de caminos (control lineal)/Cálculo de parámetros/Subsystem ==
  x_camino : Inport  Port=1  PortWidth=-1  SampleTime=-1  DataType=auto
      settings: SignalType=auto
  y_camino : Inport  Port=2  PortWidth=-1  SampleTime=-1  DataType=auto
      settings: SignalType=auto
  x_vehiculo : Inport  Port=3  PortWidth=-1  SampleTime=-1  DataType=auto
      settings: SignalType=auto
  y_vehiculo : Inport  Port=4  PortWidth=-1  SampleTime=-1  DataType=auto
      settings: SignalType=auto
  Parametros de Curvatura : Subsystem
  Product : Product  Inputs=2  SaturateOnIntegerOverflow=on
  Rc - dist : Sum  Inputs=-+  SaturateOnIntegerOverflow=on
  Sign : Signum
  Subsystem : Subsystem
  distancia mínima1 : Subsystem
  tres_puntos : Subsystem
  distancia : Outport  Port=1
  indice : Outport  Port=2
  R_c : Outport  Port=3
  wires:
  Rc - dist/1 -> Sign/1
  Subsystem/1(dist) -> Rc - dist/1
  Parametros de Curvatura/2(y_g) -> Subsystem/4(y_g)
  Parametros de Curvatura/1(x_g) -> Subsystem/3(x_g)
  Sign/1 -> Product/1
  distancia mínima1/1(d_min) -> Product/2
  tres_puntos/2(x_2) -> Parametros de Curvatura/2(x_2)
  tres_puntos/3(x_3) -> Parametros de Curvatura/3(x_3)
  tres_puntos/5(y_2) -> Parametros de Curvatura/5(y_2)
  tres_puntos/6(y_3) -> Parametros de Curvatura/6(y_3)
  x_camino/1 -> distancia mínima1/1(x_camino)
  y_camino/1 -> distancia mínima1/2(y_camino)
  Product/1 -> distancia/1
  tres_puntos/1(x_1) -> Parametros de Curvatura/1(x_1)
  tres_puntos/4(y_1) -> Parametros de Curvatura/4(y_1)
  x_vehiculo/1 -> distancia mínima1/3(x_vehiculo), Subsystem/1(x)
  y_vehiculo/1 -> distancia mínima1/4(y_vehiculo), Subsystem/2(y)
  Parametros de Curvatura/3(R_c) -> Rc - dist/2, R_c/1
  distancia mínima1/2(indice) -> indice/1, tres_puntos/1(indice)

== system HEMERO/Robots móviles/Control de robots móviles/Métodos basados en Teoría de Control/Seguimiento de caminos/Seguimiento de caminos (control no lineal)/Cálculo de parámetros/Cálculo de phi gorro ==
  fi_vehiculo : Inport  Port=1  PortWidth=-1  SampleTime=-1  DataType=auto
      settings: SignalType=auto
  indice : Inport  Port=2  PortWidth=-1  SampleTime=-1  DataType=auto
      settings: SignalType=auto
  Subsystem : Subsystem
      mask Type: Pasa phi a un ángulo entre -180 y 180
      mask Description: Pasa phi a un ángulo entre -180 y 180
      mask Help: Pasa phi a un ángulo entre -180 y 180
  Subsystem1 : Subsystem
  Subsystem2 : Subsystem
      mask Description: Pasa phi gorro al intervalo -180,180
  suma : Sum  Inputs=+-  SaturateOnIntegerOverflow=on
  fi_go_mo : Outport  Port=1
  wires:
  Subsystem2/1(fi_go_mo) -> fi_go_mo/1
  suma/1 -> Subsystem2/1(fi_gorro)
  Subsystem/1(fi_veh_mod) -> suma/1
  indice/1 -> Subsystem1/1(indice)
  fi_vehiculo/1 -> Subsystem/1(fi_vehiculo)
  Subsystem1/1(fi_camino) -> suma/2

== system HEMERO/Robots móviles/Control de robots móviles/Métodos basados en Teoría de Control/Seguimiento de caminos/Seguimiento de caminos (control no lineal)/Cálculo de parámetros/Subsystem ==
  x_camino : Inport  Port=1  PortWidth=-1  SampleTime=-1  DataType=auto
      settings: SignalType=auto
  y_camino : Inport  Port=2  PortWidth=-1  SampleTime=-1  DataType=auto
      settings: SignalType=auto
  x_vehiculo : Inport  Port=3  PortWidth=-1  SampleTime=-1  DataType=auto
      settings: SignalType=auto
  y_vehiculo : Inport  Port=4  PortWidth=-1  SampleTime=-1  DataType=auto
      settings: SignalType=auto
  Parametros de Curvatura : Subsystem
  Product : Product  Inputs=2  SaturateOnIntegerOverflow=on
  Rc - dist : Sum  Inputs=-+  SaturateOnIntegerOverflow=on
  Sign : Signum
  Subsystem : Subsystem
  distancia mínima1 : Subsystem
  tres_puntos : Subsystem
  distancia : Outport  Port=1
  indice : Outport  Port=2
  R_c : Outport  Port=3
  wires:
  distancia mínima1/2(indice) -> tres_puntos/1(indice), indice/1
  Parametros de Curvatura/3(R_c) -> R_c/1, Rc - dist/2
  y_vehiculo/1 -> Subsystem/2(y), distancia mínima1/4(y_vehiculo)
  x_vehiculo/1 -> Subsystem/1(x), distancia mínima1/3(x_vehiculo)
  tres_puntos/4(y_1) -> Parametros de Curvatura/4(y_1)
  tres_puntos/1(x_1) -> Parametros de Curvatura/1(x_1)
  Product/1 -> distancia/1
  y_camino/1 -> distancia mínima1/2(y_camino)
  x_camino/1 -> distancia mínima1/1(x_camino)
  tres_puntos/6(y_3) -> Parametros de Curvatura/6(y_3)
  tres_puntos/5(y_2) -> Parametros de Curvatura/5(y_2)
  tres_puntos/3(x_3) -> Parametros de Curvatura/3(x_3)
  tres_puntos/2(x_2) -> Parametros de Curvatura/2(x_2)
  distancia mínima1/1(d_min) -> Product/2
  Sign/1 -> Product/1
  Parametros de Curvatura/1(x_g) -> Subsystem/3(x_g)
  Parametros de Curvatura/2(y_g) -> Subsystem/4(y_g)
  Subsystem/1(dist) -> Rc - dist/1
  Rc - dist/1 -> Sign/1
